simulink model "myproject_task"  (Simulink 3.00)
undefined symbols (not defined in the file): Byte, dmstart, dmstop, dstart, dstop, perf, period, start, stop, tavg, tlast, tmax, tmin, tmover, U8
libraries: mathlib x41, paramlib x13, REXduino_library x5, logiclib x4, arclib x4, genlib x2, analoglib x2, matrixlib x1

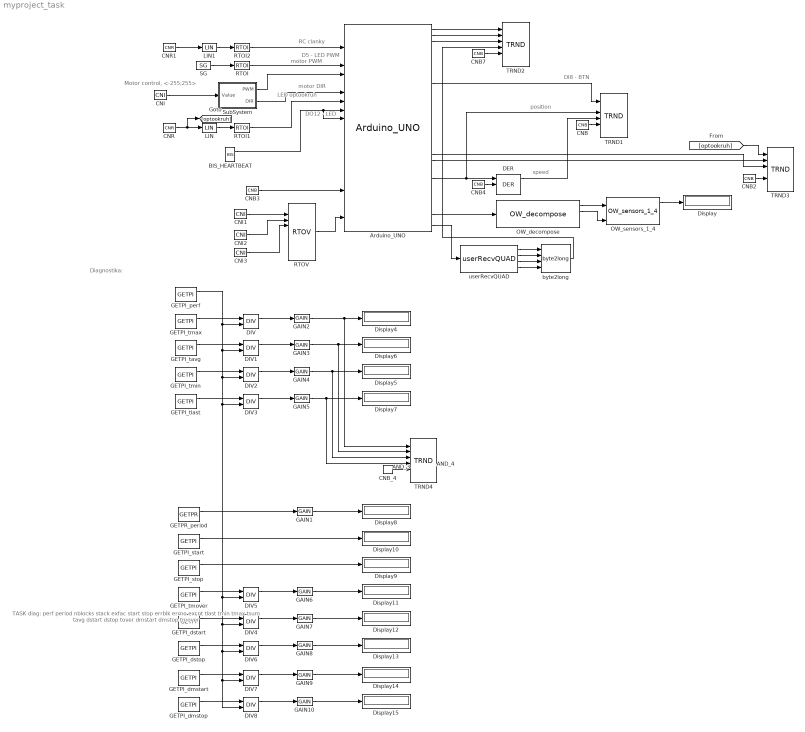
== system myproject_task ==
  note: DO12 - LED
  note: Motor control, <-255;255>
  note: D5 - LED PWM
  note: DI8 - BTN
  note: position
  note: speed
  note: motor PWM
  note: motor DIR
  note: LED optookruh
  note: RC clanky
  note: TASK diag:
      | perf
      | period
      | nblocks
      | stack
      | exfac
      | start
      | stop
      | errblk
      | errno
      | excnt
      | tlast
      | tmin
      | tmax
      | tsum
      | tavg
      | dstart
      | dstop
      | tover
      | dmstart
      | dmstop
      | tmover
  note: Diagnostika:
  AND_3 : logiclib/AND_
  AND_4 : logiclib/AND_
  Arduino_UNO : REXduino_library/Arduino_UNO  comPort=/dev/ttyACM0  pinmode2=9: Encoder A  pinmode3=1: Not connected  pinmode4=10: Counter DIR / Encoder B  pinmode5=5: PWM (analog output)  pinmode6=5: PWM (analog output)  pinmode9=1: Not connected  pinmode10=2: Digital output  pinmode11=5: PWM (analog output)  pinmodeA0=1: Not connected  pinmodeA1=1: Not connected  pinmodeA2=6: Analog input  pinmodeA3=6: Analog input  pinmodeA4=1: Not connected  pinmodeA5=1: Not connected  usercmd=2: Four bytes
  BIS_HEARTBEAT : genlib/BIS  Y0=off  t1=0.7  t2=0.8  t3=0.9  t4=1.0  t5=0  t6=6  t7=7  t8=8  RPT=on
  CNB{,2..4,7} (5 alike) : mathlib/CNB  YCN=on
  CNB_4 : mathlib/CNB  YCN=on
  CNI : mathlib/CNI  icn=0
  CNI1 : mathlib/CNI  icn=0
  CNI2 : mathlib/CNI  icn=1
  CNI3 : mathlib/CNI  icn=0x77CC
  CNR : mathlib/CNR  ycn=0
  CNR1 : mathlib/CNR  ycn=0
  DER : analoglib/DER  n=20  nmax=1000
  DIV{,1..8} (9 alike) : mathlib/DIV  yerr=0
  Display{,4..15} (13 alike) : Display
      Display settings: Format=Best fit  Suffix=??C
      Display10 settings: Format=Best fit
      Display11 settings: Format=short  Suffix=ms
      Display12 settings: Format=short  Suffix=ms
      Display13 settings: Format=short  Suffix=ms
      Display14 settings: Format=short  Suffix=ms
      Display15 settings: Format=short  Suffix=ms
      Display4 settings: Format=short  Suffix=ms
      Display5 settings: Format=short  Suffix=ms
      Display6 settings: Format=short  Suffix=ms
      Display7 settings: Format=short  Suffix=ms
      Display8 settings: Format=short  Suffix=ms
      Display9 settings: Format=Best fit
  GAIN{1..10} (10 alike) : mathlib/GAIN  k=1000
  GETPI_dmstart : paramlib/GETPI  sc=.:dmstart  GETF=off
  GETPI_dmstop : paramlib/GETPI  sc=.:dmstop  GETF=off
  GETPI_dstart : paramlib/GETPI  sc=.:dstart  GETF=off
  GETPI_dstop : paramlib/GETPI  sc=.:dstop  GETF=off
  GETPI_perf : paramlib/GETPI  sc=.:perf  GETF=off
  GETPI_start : paramlib/GETPI  sc=.:start  GETF=off
  GETPI_stop : paramlib/GETPI  sc=.:stop  GETF=off
  GETPI_tavg : paramlib/GETPI  sc=.:tavg  GETF=off
  GETPI_tlast : paramlib/GETPI  sc=.:tlast  GETF=off
  GETPI_tmax : paramlib/GETPI  sc=.:tmax  GETF=off
  GETPI_tmin : paramlib/GETPI  sc=.:tmin  GETF=off
  GETPI_tmover : paramlib/GETPI  sc=.:tmover  GETF=off
  GETPR_period : paramlib/GETPR  sc=.:period  GETF=off
  LIN : mathlib/LIN  u1=0  y1=0  u2=1  y2=255
  LIN1 : mathlib/LIN  u1=0  y1=0  u2=1  y2=255
  OW_decompose : REXduino_library/OW_decompose
      mask Type: REX sequence
  OW_sensors_1_4 : REXduino_library/OW_sensors_1_4
      mask Type: REX sequence
  RTOI : mathlib/RTOI
  RTOI1 : mathlib/RTOI
  RTOI2 : mathlib/RTOI
  RTOV : matrixlib/RTOV  nmax=16  offset=0  n=8  etype=2: Byte (U8)
  SG : genlib/SG  isig=3: SAWTOOTH  amp=50  freq=0.2  phase=0  offset=50  ifrunit=1: Hz  iphunit=1: degrees
  SubSystem : Subsystem
      mask Type: REX sequence
  TRND1 : arclib/TRND  n=4  l=1000  btype=8: Double  ptype1=1: Store  ptype2=1: Store  ptype3=1: Store  ptype4=1: Store  pfac=1  afac=0  arc=0  id=0  Title=Trend Title  timesrc=1: CORETIMER
  TRND2 : arclib/TRND  n=4  l=1000  btype=8: Double  ptype1=1: Store  ptype2=1: Store  ptype3=1: Store  ptype4=1: Store  pfac=1  afac=0  arc=0  id=0  Title=Trend Title  timesrc=1: CORETIMER
  TRND3 : arclib/TRND  n=4  l=1000  btype=8: Double  ptype1=1: Store  ptype2=1: Store  ptype3=1: Store  ptype4=1: Store  pfac=1  afac=0  arc=0  id=0  Title=Trend Title  timesrc=1: CORETIMER
  TRND4 : arclib/TRND  n=4  l=15000  btype=8: Double  ptype1=1: Store  ptype2=1: Store  ptype3=1: Store  ptype4=1: Store  pfac=1  afac=0  arc=0  id=1  Title=Execution times  timesrc=3: RTC
  byte2long : REXduino_library/byte2long
      mask Type: REX sequence
  userRecvQUAD : REXduino_library/userRecvQUAD
      mask Type: REX sequence
  wires:
  Arduino_UNO/1 -> TRND2/1
  Arduino_UNO/2 -> TRND2/2
  Arduino_UNO/3 -> TRND2/3
  Arduino_UNO/10 -> TRND1/1
  Arduino_UNO/22 -> TRND3/3
  Arduino_UNO/23 -> TRND3/2
  Arduino_UNO/26 -> DER/1, TRND1/3
  Arduino_UNO/32 -> OW_decompose/1
  Arduino_UNO/34 -> userRecvQUAD/1
  BIS_HEARTBEAT/1 -> Arduino_UNO/9, Arduino_UNO/10
  CNB/1 -> TRND1/5
  CNB2/1 -> TRND3/5
  CNB3/1 -> Arduino_UNO/18
  CNB4/1 -> DER/2
  CNB7/1 -> TRND2/5
  CNB_4/1 -> TRND4/5
  CNI/1 -> SubSystem/1(Value)
  CNI1/1 -> RTOV/2
  CNI2/1 -> RTOV/3
  CNI3/1 -> RTOV/4
  CNR/1 -> [optookruh], LIN/1
  CNR1/1 -> LIN1/1
  DER/1 -> TRND1/4
  DIV/1 -> GAIN2/1
  DIV1/1 -> GAIN3/1
  DIV2/1 -> GAIN4/1
  DIV3/1 -> GAIN5/1
  DIV4/1 -> GAIN7/1
  DIV5/1 -> GAIN6/1
  DIV6/1 -> GAIN8/1
  DIV7/1 -> GAIN9/1
  DIV8/1 -> GAIN10/1
  [optookruh] -> TRND3/1
  GAIN1/1 -> Display8/1
  GAIN10/1 -> Display15/1
  GAIN2/1 -> Display4/1, TRND4/1
  GAIN3/1 -> Display6/1, TRND4/2
  GAIN4/1 -> Display5/1, TRND4/3
  GAIN5/1 -> Display7/1, TRND4/4
  GAIN6/1 -> Display11/1
  GAIN7/1 -> Display12/1
  GAIN8/1 -> Display13/1
  GAIN9/1 -> Display14/1
  GETPI_dmstart/1 -> DIV7/1
  GETPI_dmstop/1 -> DIV8/1
  GETPI_dstart/1 -> DIV4/1
  GETPI_dstop/1 -> DIV6/1
  GETPI_perf/1 -> DIV/2, DIV1/2, DIV2/2, DIV3/2, DIV5/2, DIV4/2, DIV6/2, DIV7/2, DIV8/2
  GETPI_start/1 -> Display10/1
  GETPI_stop/1 -> Display9/1
  GETPI_tavg/1 -> DIV1/1
  GETPI_tlast/1 -> DIV3/1
  GETPI_tmax/1 -> DIV/1
  GETPI_tmin/1 -> DIV2/1
  GETPI_tmover/1 -> DIV5/1
  GETPR_period/1 -> GAIN1/1
  LIN/1 -> RTOI1/1
  LIN1/1 -> RTOI2/1
  OW_decompose/1 -> OW_sensors_1_4/1
  OW_decompose/2 -> OW_sensors_1_4/2
  OW_sensors_1_4/1 -> Display/1
  RTOI/1 -> Arduino_UNO/4
  RTOI1/1 -> Arduino_UNO/8
  RTOI2/1 -> Arduino_UNO/2
  RTOV/1 -> Arduino_UNO/21
  SG/1 -> RTOI/1
  SubSystem/1(PWM) -> Arduino_UNO/5
  SubSystem/2(DIR) -> Arduino_UNO/7
  byte2long/1 -> TRND2/4
  userRecvQUAD/1 -> byte2long/1
  userRecvQUAD/2 -> byte2long/2
  userRecvQUAD/3 -> byte2long/3
  userRecvQUAD/4 -> byte2long/4

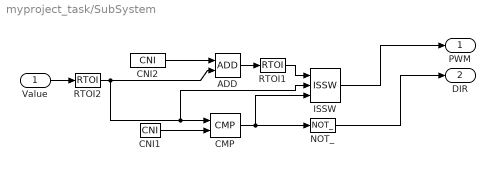
== system myproject_task/SubSystem ==
  Value : Inport  Port=1
  ADD : mathlib/ADD
  CMP : analoglib/CMP  hys=0.5
  CNI1 : mathlib/CNI  icn=0
  CNI2 : mathlib/CNI  icn=255
  ISSW : logiclib/ISSW
  NOT_ : logiclib/NOT_
  RTOI1 : mathlib/RTOI
  RTOI2 : mathlib/RTOI
  PWM : Outport  Port=1
  DIR : Outport  Port=2
  wires:
  ADD/1 -> RTOI1/1
  CMP/1 -> ISSW/3, NOT_/1
  CNI1/1 -> CMP/2
  CNI2/1 -> ADD/1
  ISSW/1 -> PWM/1
  NOT_/1 -> DIR/1
  RTOI1/1 -> ISSW/1
  RTOI2/1 -> CMP/1, ISSW/2, ADD/2
  Value/1 -> RTOI2/1
